simulink model "gm_Fixed"  (R2022b)
settings: Solver=FixedStepAuto  StartTime=0.0  StopTime=20  RelTol=1e-3
settings Model: Creator=sakyu  LastModifiedBy=sakyu
settings OptimizationCC: BlockReduction=off  ConditionallyExecuteInputs=off
settings DebuggingCC: InheritedTsInSrcMsg=none

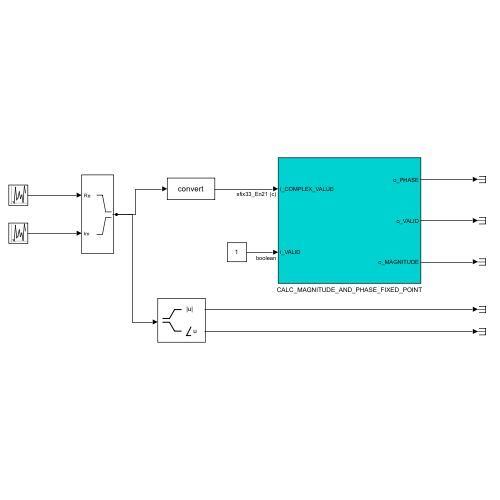
[thumbnail: Simulink's stored preview of the top-level diagram]
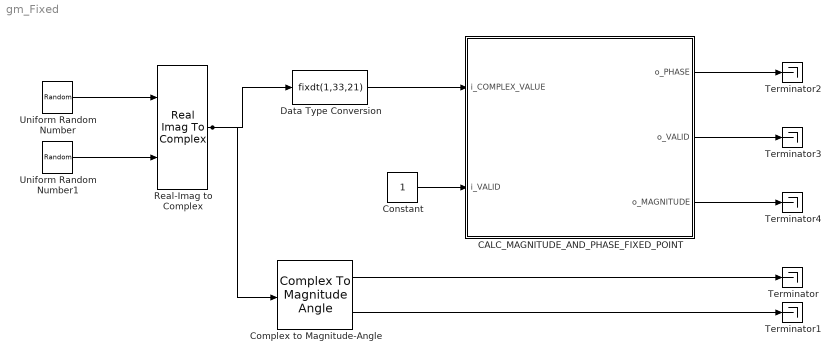
== system gm_Fixed ==
  CALC_MAGNITUDE_AND_PHASE_FIXED_POINT : Subsystem
  Complex to Magnitude-Angle : ComplexToMagnitudeAngle
  Constant : Constant  OutDataTypeStr=boolean  SampleTime=1
  Data Type Conversion : DataTypeConversion  OutDataTypeStr=fixdt(1,33,21)  RndMeth=Round  SaturateOnIntegerOverflow=off
  Real-Imag to Complex : RealImagToComplex
  Terminator{,1..4} (5 alike) : Terminator
  Uniform Random Number : UniformRandomNumber  Minimum=0  Maximum=2047.99999904632568359375  Seed=11  SampleTime=1
  Uniform Random Number1 : UniformRandomNumber  Minimum=0  Maximum=2047.999999523162841796875  Seed=12  SampleTime=1
  wires:
  CALC_MAGNITUDE_AND_PHASE_FIXED_POINT/1(o_PHASE) -> Terminator2/1
  CALC_MAGNITUDE_AND_PHASE_FIXED_POINT/2(o_VALID) -> Terminator3/1
  CALC_MAGNITUDE_AND_PHASE_FIXED_POINT/3(o_MAGNITUDE) -> Terminator4/1
  Constant/1 -> CALC_MAGNITUDE_AND_PHASE_FIXED_POINT/2(i_VALID)
  Data Type Conversion/1 -> CALC_MAGNITUDE_AND_PHASE_FIXED_POINT/1(i_COMPLEX_VALUE)
  Complex to Magnitude-Angle/2 -> Terminator1/1
  Complex to Magnitude-Angle/1 -> Terminator/1
  Real-Imag to Complex/1 -> Data Type Conversion/1, Complex to Magnitude-Angle/1
  Uniform Random Number1/1 -> Real-Imag to Complex/2
  Uniform Random Number/1 -> Real-Imag to Complex/1

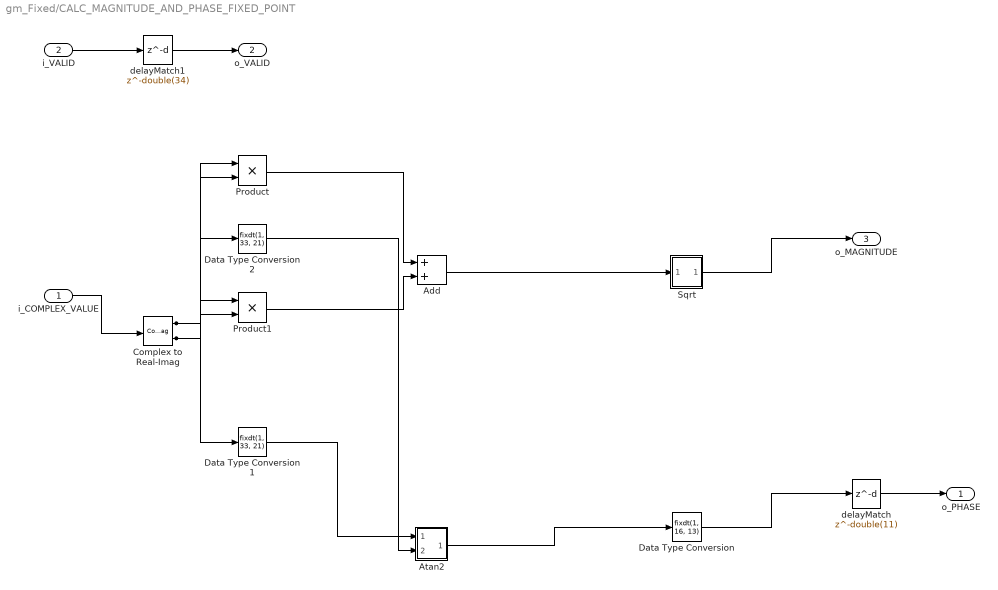
== system gm_Fixed/CALC_MAGNITUDE_AND_PHASE_FIXED_POINT ==
  i_COMPLEX_VALUE : Inport  OutDataTypeStr=fixdt(1, 33, 21)  PortDimensions=1  SampleTime=1
      settings: SignalType=complex
  i_VALID : Inport  Port=2  OutDataTypeStr=boolean  PortDimensions=1  SampleTime=1
  Add : Sum  AccumDataTypeStr=fixdt(1, 66, 42)  OutDataTypeStr=fixdt(1, 66, 42)  SampleTime=1
  Atan2 : Subsystem
  Complex to Real-Imag : ComplexToRealImag  SampleTime=1
  Data Type Conversion : DataTypeConversion  OutDataTypeStr=fixdt(1, 16, 13)  SampleTime=1  SaturateOnIntegerOverflow=off  RndMeth=Floor
  Data Type Conversion1 : DataTypeConversion  OutDataTypeStr=fixdt(1, 33, 21)  SampleTime=1  SaturateOnIntegerOverflow=off  RndMeth=Floor
  Data Type Conversion2 : DataTypeConversion  OutDataTypeStr=fixdt(1, 33, 21)  SampleTime=1  SaturateOnIntegerOverflow=off  RndMeth=Floor
  Product : Product  Inputs=**  OutDataTypeStr=fixdt(1, 65, 42)  SampleTime=1
  Product1 : Product  Inputs=**  OutDataTypeStr=fixdt(1, 65, 42)  SampleTime=1
  Sqrt : Subsystem
  delayMatch : Delay  DelayLength=double(11)  InitialCondition=0  SampleTime=1
  delayMatch1 : Delay  DelayLength=double(34)  InitialCondition=0  SampleTime=1
  o_PHASE : Outport  SampleTime=1
  o_VALID : Outport  Port=2  SampleTime=1
  o_MAGNITUDE : Outport  Port=3  SampleTime=1
  wires:
  i_COMPLEX_VALUE/1 -> Complex to Real-Imag/1
  delayMatch1/1 -> o_VALID/1
  Add/1 -> Sqrt/1(In1)
  Atan2/1(Out1) -> Data Type Conversion/1
  Complex to Real-Imag/1 -> Data Type Conversion2/1, Product/2, Product/1
  Complex to Real-Imag/2 -> Data Type Conversion1/1, Product1/2, Product1/1
  delayMatch/1 -> o_PHASE/1
  Data Type Conversion1/1 -> Atan2/1(In1)
  Data Type Conversion2/1 -> Atan2/2(In2)
  Product/1 -> Add/1
  Product1/1 -> Add/2
  Sqrt/1(Out1) -> o_MAGNITUDE/1
  Data Type Conversion/1 -> delayMatch/1
  i_VALID/1 -> delayMatch1/1

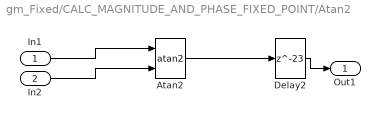
== system gm_Fixed/CALC_MAGNITUDE_AND_PHASE_FIXED_POINT/Atan2 ==
  In1 : Inport
  In2 : Inport  Port=2
  Atan2 : Trigonometry  Operator=atan2  ApproximationMethod=CORDIC  NumberOfIterations=20
  Delay2 : Delay  DelayLength=23
  Out1 : Outport
  wires:
  In1/1 -> Atan2/1
  In2/1 -> Atan2/2
  Atan2/1 -> Delay2/1
  Delay2/1 -> Out1/1

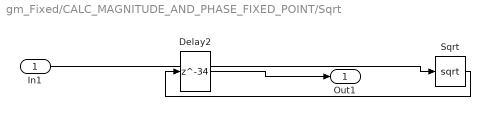
== system gm_Fixed/CALC_MAGNITUDE_AND_PHASE_FIXED_POINT/Sqrt ==
  In1 : Inport
  Delay2 : Delay  DelayLength=34
  Sqrt : Sqrt  OutDataTypeStr=fixdt(1,33,21)
  Out1 : Outport
  wires:
  In1/1 -> Sqrt/1
  Sqrt/1 -> Delay2/1
  Delay2/1 -> Out1/1
